simulink model "MyBatteryCU_RTW"  (Simulink 10.1)
settings: Solver=ode1  StartTime=0.0  StopTime=inf  FixedStep=0.0002  RelTol=1e-3
PreLoadFcn:
  | vehicle = 'Car'; if ~length(which('cmself')), cmenv; end
  | MyBatteryCU_RTW_bus
InitFcn:
  | vehicle = 'Car'; if ~length(which('cmself')), cmenv; end
  | MyBatteryCU_RTW_bus
Description:
  | CarMaker Plug-in Model Target
settings Model: Creator=ml  LastModifiedBy=ml
settings DataIOCC: SaveFormat=Dataset  ReturnWorkspaceOutputs=on
settings OptimizationCC: LifeSpan=auto
settings DebuggingCC: UnderspecifiedInitializationDetection=Simplified  MergeDetectMultiDrivingBlocksExec=error  SFUnexpectedBacktrackingDiag=error  SFNoUnconditionalDefaultTransitionDiag=error  SFExecutionAtInitializationDiag=warning  ArithmeticOperatorsInVariantConditions=error
settings HardwareCC: ProdBitPerPointer=64  ProdBitPerSizeT=64  ProdBitPerPtrDiffT=64  ProdLargestAtomicFloat=Float  ProdIntDivRoundTo=Zero  ProdEndianess=LittleEndian  ProdWordSize=64  ProdHWDeviceType=Intel->x86-64 (Windows64)
settings ModelReferenceCC: PropagateSignalLabelsOutOfModel=on
settings SFSimCC: SimUseLocalCustomCode=on  CustomCodeUndefinedFunction=FilterOut
settings RTWCC: Description=CarMaker Plug-in Model Target  SystemTargetFile=CarMaker.tlc  TemplateMakefile=CarMaker_unix-win64.tmf  RTWUseLocalCustomCode=on
settings CodeAppCC: MaxIdLength=127  StateflowObjectComments=off
settings STFCustomTargetCC: TargetLangStandard=C99 (ISO)  CombineOutputUpdateFcns=on  MultiInstanceERTCode=on  CodeInterfacePackaging=Reusable function  GRTInterface=off  GenerateAllocFcn=on  SystemTargetFile=CarMaker.tlc
settings GRTTargetCC: TargetLangStandard=C99 (ISO)  ParMdlRefBuildCompliant=off  CompOptLevelCompliant=off  ConcurrentExecutionCompliant=off  CombineOutputUpdateFcns=on  MatFileLogging=off  MultiInstanceERTCode=on  CodeInterfacePackaging=Reusable function  CPPClassGenCompliant=off  GRTInterface=off  GenerateAllocFcn=on  UseToolchainInfoCompliant=off
settings CustomProperty: DataType=string
settings EnumStrPairs: String=Car
settings ConfigComp: CovMetricSettings=dwe  CovHtmlReporting=off  CovSaveCumulativeToWorkspaceVar=off  CovSaveSingleToWorkspaceVar=off  CovExternalEMLEnable=on

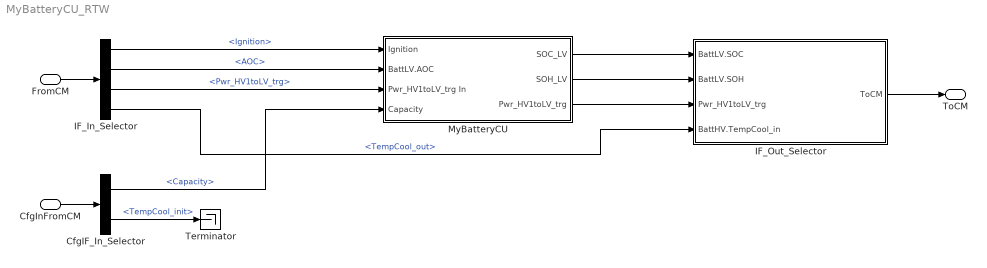
== system MyBatteryCU_RTW ==
  FromCM : Inport  OutDataTypeStr=Bus: cmPTBatteryCUIn
  CfgInFromCM : Inport  Port=2  OutDataTypeStr=Bus: cmPTBatteryCUCfgIn
  CfgIF_In_Selector : BusSelector  OutputSignals=BattLV.Capacity,BattLV.TempCool_init
  IF_In_Selector : BusSelector  OutputSignals=Ignition,BattLV.AOC,Pwr_HV1toLV_trg,BattLV.TempCool_out
  IF_Out_Selector : Subsystem  mask(Signal Selection){}
      mask help: Signal Selection Block
      settings: OpenFcn=cmSignalSelect('SignalSelection_CB',gcb)
  MyBatteryCU : Subsystem
  Terminator : Terminator
  ToCM : Outport  OutDataTypeStr=Bus: cmPTBatteryCUOut
  wires:
  IF_Out_Selector/1(ToCM) -> ToCM/1
  CfgIF_In_Selector/2 -> Terminator/1  "<TempCool_init>"
  FromCM/1 -> IF_In_Selector/1
  MyBatteryCU/2(SOH_LV) -> IF_Out_Selector/2(BattLV.SOH)
  CfgIF_In_Selector/1 -> MyBatteryCU/4(Capacity)  "<Capacity>"
  MyBatteryCU/1(SOC_LV) -> IF_Out_Selector/1(BattLV.SOC)
  IF_In_Selector/2 -> MyBatteryCU/2(BattLV.AOC)  "<AOC>"
  IF_In_Selector/1 -> MyBatteryCU/1(Ignition)  "<Ignition>"
  MyBatteryCU/3(Pwr_HV1toLV_trg) -> IF_Out_Selector/3(Pwr_HV1toLV_trg)
  IF_In_Selector/3 -> MyBatteryCU/3(Pwr_HV1toLV_trg In)  "<Pwr_HV1toLV_trg>"
  IF_In_Selector/4 -> IF_Out_Selector/4(BattHV.TempCool_in)  "<TempCool_out>"
  CfgInFromCM/1 -> CfgIF_In_Selector/1

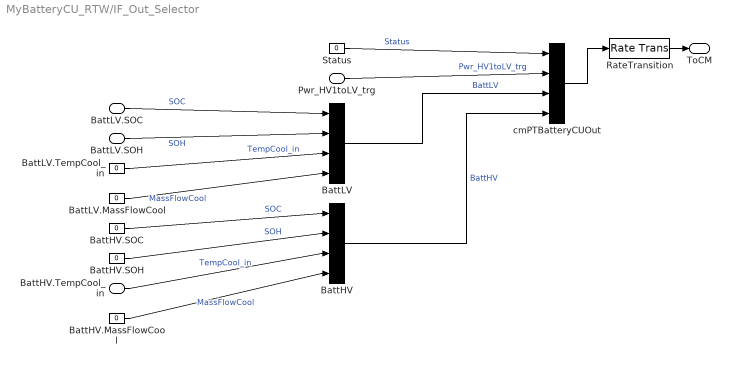
== system MyBatteryCU_RTW/IF_Out_Selector ==
  BattLV.SOC : Inport
  BattLV.SOH : Inport  Port=2
  Pwr_HV1toLV_trg : Inport  Port=3
  BattHV.TempCool_in : Inport  Port=4
  BattHV : BusCreator  Inputs=4
  BattHV.MassFlowCool : Constant  Value=0
  BattHV.SOC : Constant  Value=0
  BattHV.SOH : Constant  Value=0
  BattLV : BusCreator  Inputs=4
  BattLV.MassFlowCool : Constant  Value=0
  BattLV.TempCool_in : Constant  Value=0
  RateTransition : RateTransition  OutPortSampleTime=str2num(get_param(bdroot,'FixedStep'))
  Status : Constant  Value=0
  cmPTBatteryCUOut : BusCreator  Inputs=4
  ToCM : Outport
  wires:
  RateTransition/1 -> ToCM/1
  cmPTBatteryCUOut/1 -> RateTransition/1
  Status/1 -> cmPTBatteryCUOut/1  "Status"
  BattLV/1 -> cmPTBatteryCUOut/3  "BattLV"
  BattLV.TempCool_in/1 -> BattLV/3  "TempCool_in"
  BattLV.MassFlowCool/1 -> BattLV/4  "MassFlowCool"
  BattHV/1 -> cmPTBatteryCUOut/4  "BattHV"
  BattHV.SOC/1 -> BattHV/1  "SOC"
  BattHV.SOH/1 -> BattHV/2  "SOH"
  BattHV.MassFlowCool/1 -> BattHV/4  "MassFlowCool"
  BattLV.SOC/1 -> BattLV/1  "SOC"
  BattLV.SOH/1 -> BattLV/2  "SOH"
  Pwr_HV1toLV_trg/1 -> cmPTBatteryCUOut/2  "Pwr_HV1toLV_trg"
  BattHV.TempCool_in/1 -> BattHV/3  "TempCool_in"

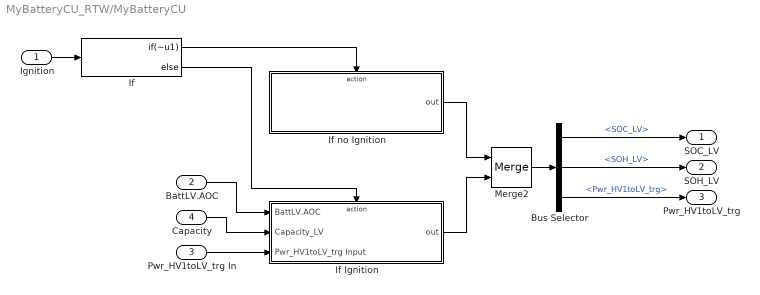
== system MyBatteryCU_RTW/MyBatteryCU ==
  Ignition : Inport
  BattLV.AOC : Inport  Port=2
  Pwr_HV1toLV_trg In : Inport  Port=3
  Capacity : Inport  Port=4
  Bus Selector : BusSelector  OutputSignals=SOC_LV,SOH_LV,Pwr_HV1toLV_trg
  If : If  IfExpression=~u1
  If Ignition : Subsystem  TreatAsAtomicUnit=on
  If no Ignition : Subsystem  TreatAsAtomicUnit=on
  Merge2 : Merge
  SOC_LV : Outport  VectorParamsAs1DForOutWhenUnconnected=off
  SOH_LV : Outport  Port=2  VectorParamsAs1DForOutWhenUnconnected=off
  Pwr_HV1toLV_trg : Outport  Port=3  VectorParamsAs1DForOutWhenUnconnected=off
  wires:
  Ignition/1 -> If/1
  If/1 -> If no Ignition/Action
  BattLV.AOC/1 -> If Ignition/1(BattLV.AOC)
  Capacity/1 -> If Ignition/2(Capacity_LV)
  Pwr_HV1toLV_trg In/1 -> If Ignition/3(Pwr_HV1toLV_trg Input)
  If/2 -> If Ignition/Action
  Merge2/1 -> Bus Selector/1
  If Ignition/1(out) -> Merge2/2
  If no Ignition/1(out) -> Merge2/1
  Bus Selector/1 -> SOC_LV/1  "<SOC_LV>"
  Bus Selector/2 -> SOH_LV/1  "<SOH_LV>"
  Bus Selector/3 -> Pwr_HV1toLV_trg/1  "<Pwr_HV1toLV_trg>"

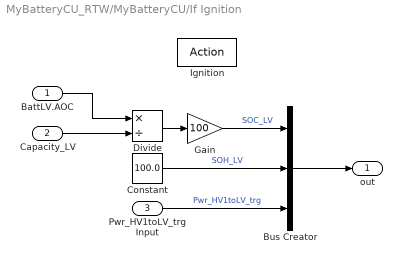
== system MyBatteryCU_RTW/MyBatteryCU/If Ignition ==
  BattLV.AOC : Inport
  Capacity_LV : Inport  Port=2
  Pwr_HV1toLV_trg Input : Inport  Port=3
  Ignition : ActionPort  ActionPortLabel=else
  Bus Creator : BusCreator  Inputs=3
  Constant : Constant  Value=100.0
  Divide : Product  Inputs=*/
  Gain : Gain  Gain=100
  out : Outport  InitialOutput=[,100,]  VectorParamsAs1DForOutWhenUnconnected=off
  wires:
  Constant/1 -> Bus Creator/2  "SOH_LV"
  BattLV.AOC/1 -> Divide/1
  Capacity_LV/1 -> Divide/2
  Divide/1 -> Gain/1
  Gain/1 -> Bus Creator/1  "SOC_LV"
  Pwr_HV1toLV_trg Input/1 -> Bus Creator/3  "Pwr_HV1toLV_trg"
  Bus Creator/1 -> out/1

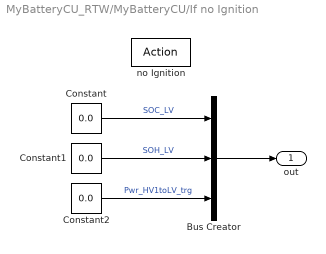
== system MyBatteryCU_RTW/MyBatteryCU/If no Ignition ==
  no Ignition : ActionPort  ActionPortLabel=if(~u1)
  Bus Creator : BusCreator  Inputs=3
  Constant : Constant  Value=0.0
  Constant1 : Constant  Value=0.0
  Constant2 : Constant  Value=0.0
  out : Outport  InitialOutput=0  VectorParamsAs1DForOutWhenUnconnected=off
  wires:
  Constant1/1 -> Bus Creator/2  "SOH_LV"
  Constant/1 -> Bus Creator/1  "SOC_LV"
  Constant2/1 -> Bus Creator/3  "Pwr_HV1toLV_trg"
  Bus Creator/1 -> out/1
